simulink model "ODE2"  (Simulink 7.8)
settings: Solver=ode45  StartTime=0.0  StopTime=10  RelTol=1e-3
undefined symbols (not defined in the file): a, b, c
settings Model: Creator=susana  LastModifiedBy=susana

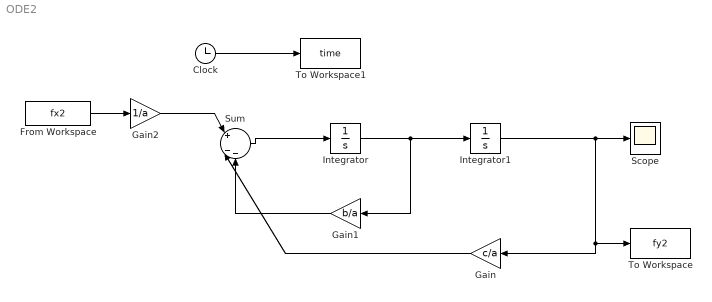
== system ODE2 ==
  Clock : Clock
  From Workspace : FromWorkspace  VariableName=fx2  SampleTime=0  OutputAfterFinalValue=Setting to zero
  Gain : Gain  Gain=c/a
  Gain1 : Gain  Gain=b/a
  Gain2 : Gain  Gain=1/a
  Integrator : Integrator
  Integrator1 : Integrator
  Scope : Scope
  Sum : Sum  Inputs=|+|--
  To Workspace : ToWorkspace  VariableName=fy2  SampleTime=-1  SaveFormat=Array
  To Workspace1 : ToWorkspace  VariableName=time  SampleTime=-1  SaveFormat=Array
  wires:
  Integrator/1 -> Integrator1/1, Gain1/1
  Integrator1/1 -> Scope/1, Gain/1, To Workspace/1
  Sum/1 -> Integrator/1
  Gain1/1 -> Sum/3
  Gain/1 -> Sum/2
  Gain2/1 -> Sum/1
  From Workspace/1 -> Gain2/1
  Clock/1 -> To Workspace1/1
